simulink model "Sistem_de_actionare_electrica_cu_motor_de_curent_continuu"  (R2022b)
settings: Solver=VariableStepAuto  StartTime=0.0  StopTime=10.0  RelTol=1e-3
values from neighbouring files (symbols this model uses):
  A = [-1/Ta -ke/La ; km/J 0]    [Sistem_de_actionare_electrica_cu_motor.m]
  B = [kE/La 0 ; 0 -1/J]    [Sistem_de_actionare_electrica_cu_motor.m]
  C = [1 0 ; 0 1]    [Sistem_de_actionare_electrica_cu_motor.m]
  D = [0 0 ; 0 0]    [Sistem_de_actionare_electrica_cu_motor.m]
  J = 0.0302    [Sistem_de_actionare_electrica_cu_motor.m]
  kE = 42.85    [Sistem_de_actionare_electrica_cu_motor.m]
  ke = 0.56    [Sistem_de_actionare_electrica_cu_motor.m]
  kf = 0    [Sistem_de_actionare_electrica_cu_motor.m]
  km = 0.55    [Sistem_de_actionare_electrica_cu_motor.m]
  Ra = 5.1    [Sistem_de_actionare_electrica_cu_motor.m]
  Ta = 0.1    [Sistem_de_actionare_electrica_cu_motor.m]
  Tm = 0.5    [Sistem_de_actionare_electrica_cu_motor.m]
settings Model: Creator=Adrian  LastModifiedBy=Adrian

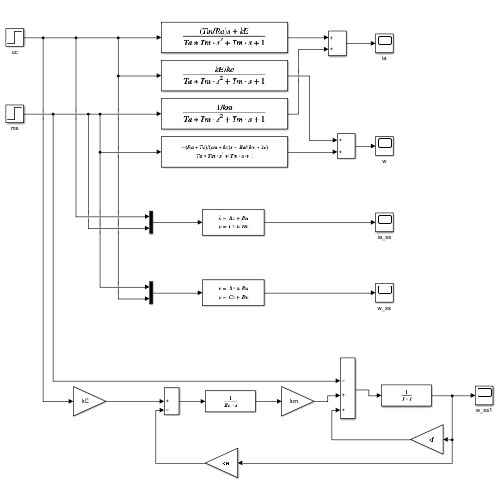
[thumbnail: Simulink's stored preview of the top-level diagram]
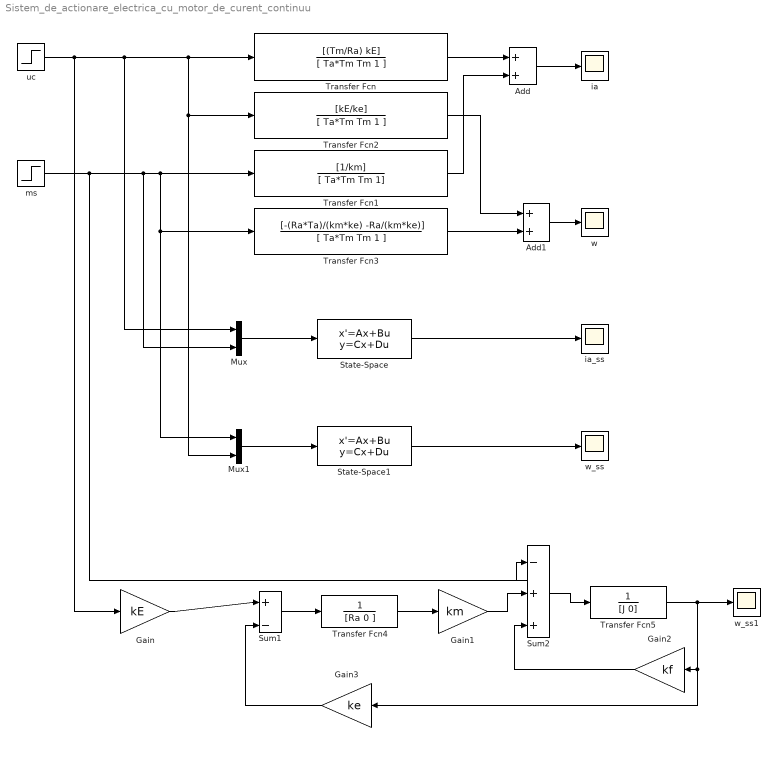
== system Sistem_de_actionare_electrica_cu_motor_de_curent_continuu ==
  Add : Sum
  Add1 : Sum
  Gain : Gain  Gain=kE
  Gain1 : Gain  Gain=km
  Gain2 : Gain  Gain=kf
  Gain3 : Gain  Gain=ke
  Mux : Mux  Inputs=2
  Mux1 : Mux  Inputs=2
  State-Space : StateSpace  A=A  B=B  C=C  D=D  InitialCondition=0
  State-Space1 : StateSpace  A=A  B=B  C=C  D=D  InitialCondition=0
  Sum1 : Sum  Inputs=|+-
  Sum2 : Sum  Inputs=|-++
  Transfer Fcn : TransferFcn  Numerator=[(Tm/Ra) kE]  Denominator=[ Ta*Tm Tm 1 ]
  Transfer Fcn1 : TransferFcn  Numerator=[1/km]  Denominator=[ Ta*Tm Tm 1]
  Transfer Fcn2 : TransferFcn  Numerator=[kE/ke]  Denominator=[ Ta*Tm Tm 1 ]
  Transfer Fcn3 : TransferFcn  Numerator=[-(Ra*Ta)/(km*ke) -Ra/(km*ke)]  Denominator=[ Ta*Tm Tm 1 ]
  Transfer Fcn4 : TransferFcn  Denominator=[Ra 0 ]
  Transfer Fcn5 : TransferFcn  Denominator=[J 0]
  ia : Scope
  ia_ss : Scope
  ms : Step  Time=0  SampleTime=0
  uc : Step  Time=0  SampleTime=0
  w : Scope
  w_ss : Scope
  w_ss1 : Scope
  wires:
  uc/1 -> Gain/1, Mux/1, Mux1/2, Transfer Fcn2/1, Transfer Fcn/1
  ms/1 -> Sum2/1, Mux/2, Transfer Fcn1/1, Mux1/1, Transfer Fcn3/1
  Transfer Fcn/1 -> Add/1
  Transfer Fcn1/1 -> Add/2
  Transfer Fcn2/1 -> Add1/1
  Transfer Fcn3/1 -> Add1/2
  Add/1 -> ia/1
  Add1/1 -> w/1
  Mux/1 -> State-Space/1
  State-Space/1 -> ia_ss/1
  Mux1/1 -> State-Space1/1
  State-Space1/1 -> w_ss/1
  Gain/1 -> Sum1/1
  Sum1/1 -> Transfer Fcn4/1
  Transfer Fcn4/1 -> Gain1/1
  Gain1/1 -> Sum2/2
  Sum2/1 -> Transfer Fcn5/1
  Transfer Fcn5/1 -> Gain3/1, Gain2/1, w_ss1/1
  Gain2/1 -> Sum2/3
  Gain3/1 -> Sum1/2
